simulink model "stock_stateflow"  (R2015b)
settings: Solver=ode45  StartTime=0.0  StopTime=10.0  RelTol=1e-3
settings Model: Creator=pound  LastModifiedBy=pound
settings DataIOCC: SaveFormat=Array
settings DebuggingCC: UnderspecifiedInitializationDetection=Classic  MergeDetectMultiDrivingBlocksExec=none  SolverPrmCheckMsg=warning
settings HardwareCC: ProdBitPerPointer=32  ProdLargestAtomicFloat=None  ProdIntDivRoundTo=Undefined  ProdEndianess=Unspecified  ProdWordSize=32  ProdHWDeviceType=32-bit Generic
settings GRTTargetCC: GeneratePreprocessorConditionals=Disable all
settings ConfigComp: CovModelRefEnable=Off

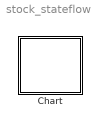
== system stock_stateflow ==
  Chart : Stateflow chart  TreatAsAtomicUnit=on

== stateflow chart stock_stateflow/Chart ==
  state Fractal_Buy
  state init
    appl[0] = 13
    appl[1] = 12
    appl[2] = 10
    appl[3] = 9
    appl[4] =  8
    appl[5] = 7
    appl[6] = 6
    appl[7] = 5
    appl[8] = 4
    appl[9] = 3
    appl[10] = 2
    appl[11] = 1
    appl[12] = 1
  state Idle
    L = 0 %Blue
    M = 0  %Red
    S = 0 %Green
    FB = 0
    FS = 1
  state Fractal_Sell
  state Sell
  state Hold
  state Buy
  (junction 75) -> Fractal_Buy [order 1] : [S > M && M > L]
  (default) -> init
  (junction 55) -> (junction 55) [order 1] : [i > 3]{L = L + appl[i];...
      |           M = M + appl[i];...
      |           i--;}
  Idle -> (junction 53) : {i=12;}
  (junction 56) -> (junction 75) [order 2] : {S = S/5.0;...
      | M = M/8.0;...
      | L = L/13.0;}
  (junction 55) -> (junction 56) [order 2]
  (junction 53) -> (junction 55) [order 2]
  (junction 75) -> Fractal_Sell [order 2] : [L > M && M > S]
  (junction 56) -> (junction 56) [order 1] : [i>=0]{L = L + appl[i]; i--}
  (junction 53) -> (junction 53) [order 1] : [i > 7]{L = L + appl[i];...
      |         M = M + appl[i];...
      |         S = S + appl[i];...
      |         i--;}
  (junction 75) -> Hold [order 3]
  init -> Idle
  Fractal_Buy -> Hold [order 1] : [!FB]
  Fractal_Buy -> Buy [order 2] : [FB]
  Buy -> Idle
  Hold -> Idle
  Sell -> Idle
  Fractal_Sell -> Sell [order 1] : [FS]
  Fractal_Sell -> Hold [order 2] : [!FS]
  data: FB local double; FS local double; L local double; M local double; S local double; appl local double size=13; i local double; sum local double
